simulink model "Scenario_PTF_path_following_v1"  (R2024b)
settings: Solver=ode1  StartTime=0.0  StopTime=1000  FixedStep=.05  RelTol=1e-3  EnableMultiTasking=on
InitFcn:
  | omega_n = 1; r_limit = 10; scale = 1;
values from neighbouring files (symbols this model uses):
  complete_Cx = B_fine * control_points    [MCM_v4.m]
  complete_DCx = B_fine * control_points_deriv    [MCM_v4.m]
  complete_time = [complete_time(1:end-1,:); segment_time_shifted']    [MCM_v4.m]
libraries: simulink x5
settings Model: Creator=isaackaminer  LastModifiedBy=bradenzukowski
settings SolverCC: AlgebraicLoopSolver=TrustRegion
settings DataIOCC: LimitDataPoints=on  SaveFormat=StructureWithTime  SignalLoggingSaveFormat=ModelDataLogs  ReturnWorkspaceOutputs=off
settings OptimizationCC: BlockReduction=off  DefaultParameterBehavior=Inlined  BufferReuse=off  LifeSpan=inf
settings DebuggingCC: SolverPrmCheckMsg=warning  MultiTaskDSMMsg=warning  MultiTaskCondExecSysMsg=none  UnconnectedInputMsg=warning  UnconnectedOutputMsg=warning  UnconnectedLineMsg=warning  InitInArrayFormatMsg=none  SFUnexpectedBacktrackingDiag=warning  SFNoUnconditionalDefaultTransitionDiag=warning  SFExecutionAtInitializationDiag=none  ArithmeticOperatorsInVariantConditions=warning
settings HardwareCC: ProdBitPerPointer=32  ProdBitPerSizeT=32  ProdBitPerPtrDiffT=32  ProdLargestAtomicFloat=None  ProdIntDivRoundTo=Undefined  ProdEndianess=Unspecified  ProdWordSize=32  ProdHWDeviceType=32-bit Generic
settings ModelReferenceCC: EnableRefExpFcnMdlSchedulingChecks=on  PropagateSignalLabelsOutOfModel=off
settings SFSimCC: SimUseLocalCustomCode=off  CustomCodeUndefinedFunction=UseInterfaceOnly
settings RTWCC: RTWUseLocalCustomCode=off  GPUComputeCapability=3.5
settings CodeAppCC: StateflowObjectComments=on
settings GRTTargetCC: TargetLangStandard=C89/C90 (ANSI)
settings ConfigComp: CovMetricSettings=dw  CovSaveCumulativeToWorkspaceVar=on  CovSaveSingleToWorkspaceVar=on  CovExternalEMLEnable=off

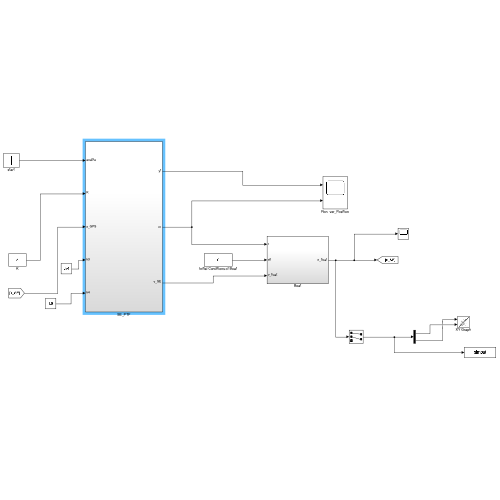
[thumbnail: Simulink's stored preview of the top-level diagram]
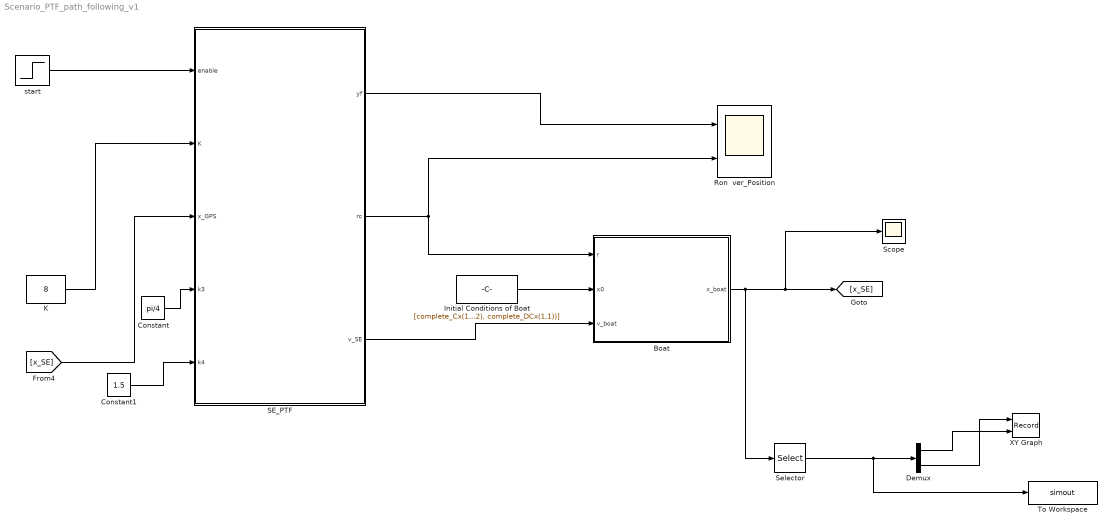
== system Scenario_PTF_path_following_v1 ==
  Boat : Subsystem
  Constant : Constant  Value=pi/4
  Constant1 : Constant  Value=1.5
  Demux : Demux  Outputs=2
  Initial Conditions of Boat : Constant  Value=[complete_Cx(1,1);complete_Cx(1,2);atan2(complete_DCx(1,2), complete_DCx(1,1))]
  K : Constant  Value=8
  Ron  ver_Position : Scope  NumInputPorts=2
  SE_PTF : Subsystem
  Scope : Scope
  Selector : Selector  InputPortWidth=3  IndexOptions=Index vector (dialog)  Indices=[1 2]  OutputSizes=1
  To Workspace : ToWorkspace  VariableName=simout  SaveFormat=Timeseries  SampleTime=-1
  XY Graph : Record  FileSettingsInternal="{\"entries\":[{\"content\":{\"excelSettings\":{\"content\":{},\"type\":\"Streamout.ExcelSettings\"}},\"type\":\"Streamout.FileSettingStorage\",\"uuid\":\"\"}],\"packageUris\":[\"http:\\/\\/schema.mathworks.com\\/mf0\\/streamout_blocks\\/R2020a\"],\"version\":\"1.0\"}"  Layout=[1 1]  SignalsInternal="{\"entries\":[{\"content\":{\"signals\":[{\"content\":{\"blockPath\":[],\"dimensions\":[1],\"domain\":\"\",\"lineColor\":\"#a2142f\",\"plots\":[ 1 ],\"port\":1,\"sid\":[\"\"],\"signalID\":1,\"signalName\":\"Demux:2\"},\"type\":\"RecordBlkView.Signal\",\"uuid\":\"\"},{\"content\":{\"blockPath\":[],\"dimensions\":[1],\"domain\":\"\",\"lineColor\":\"#139fff\",\"plots\":[ 1 ],\"port\":2,\"sid\":[\"\"],\"signalID\":2,\"signalName\":\"Demux:1\"},\"type\":\"RecordBlkView.Signal\",\"uuid\":\"\"}]},\"type\":\"RecordBlkView.InputSignals\",\"uuid\":\"\"}],\"packageUris\":[\"http:\\/\\/schema.mathworks.com\\/mf0\\/streamout_blocks\\/R2020a\"],\"version\":\"1.0\"}"  VisualizationBindings="{\"xyplotplugin\":{\"info\":[{\"series\":[{\"bindingParametersList\":[{\"parameter\":\"X-Axis\",\"signalID\":1,\"signalName\":\"Demux:2\"},{\"parameter\":\"Y-Axis\",\"signalID\":2,\"signalName\":\"Demux:1\"}],\"seriesID\":0}],\"subplotID\":1}]}}"  CompatibilityTag=XY
  start : Step  Time=0  SampleTime=0
  wires:
  start/1 -> SE_PTF/1(enable)
  SE_PTF/2(rc) -> Boat/1(r), Ron  ver_Position/2
  [x_SE] -> SE_PTF/3(x_GPS)
  SE_PTF/1(yf) -> Ron  ver_Position/1
  Demux/2 -> XY Graph/1
  Boat/1(x_boat) -> Scope/1, [x_SE], Selector/1
  Initial Conditions of Boat/1 -> Boat/2(x0)
  Selector/1 -> To Workspace/1, Demux/1
  Demux/1 -> XY Graph/2
  K/1 -> SE_PTF/2(K)
  Constant/1 -> SE_PTF/4(k3)
  Constant1/1 -> SE_PTF/5(k4)
  SE_PTF/3(v_SE) -> Boat/3(v_boat)

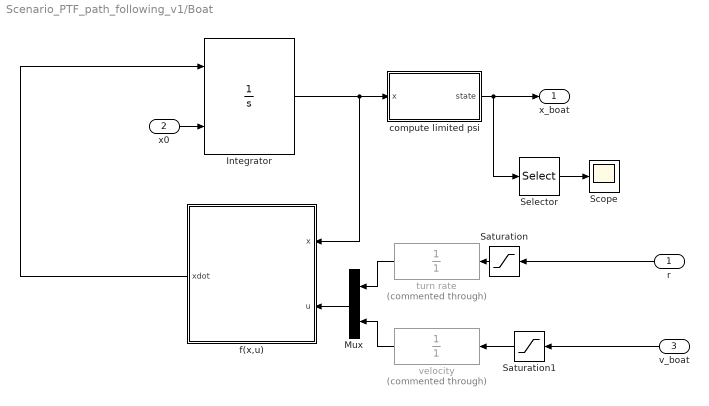
== system Scenario_PTF_path_following_v1/Boat ==
  r : Inport
  x0 : Inport  Port=2
  v_boat : Inport  Port=3
  Integrator : Integrator  InitialConditionSource=external
  Mux : Mux  Inputs=2
  Saturation : Saturate  UpperLimit=.5  LowerLimit=-.5
  Saturation1 : Saturate  UpperLimit=3  LowerLimit=0
  Scope : Scope
  Selector : Selector  InputPortWidth=3  IndexOptions=Index vector (dialog)  Indices=3  OutputSizes=1
  compute limited psi : MATLAB Function  TreatAsAtomicUnit=on
  f(x,u) : MATLAB Function  TreatAsAtomicUnit=on
  turn rate : TransferFcn  Commented=through  Denominator=[1]
  velocity : TransferFcn  Commented=through  Denominator=[1]
  x_boat : Outport  VectorParamsAs1DForOutWhenUnconnected=off
  wires:
  f(x,u)/1(xdot) -> Integrator/1
  x0/1 -> Integrator/2
  Integrator/1 -> compute limited psi/1(x), f(x,u)/1(x)
  compute limited psi/1(state) -> Selector/1, x_boat/1
  turn rate/1 -> Mux/1
  Mux/1 -> f(x,u)/2(u)
  Selector/1 -> Scope/1
  velocity/1 -> Mux/2
  Saturation/1 -> turn rate/1
  r/1 -> Saturation/1
  Saturation1/1 -> velocity/1
  v_boat/1 -> Saturation1/1

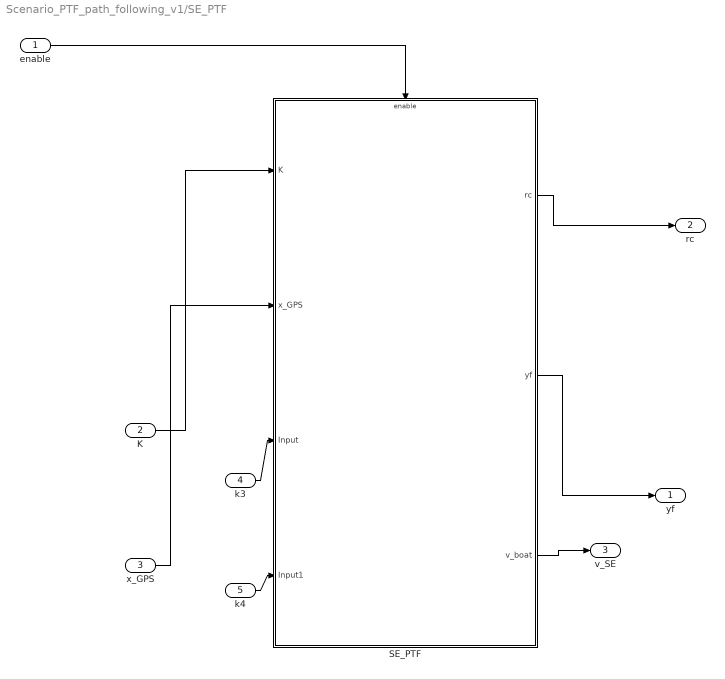
== system Scenario_PTF_path_following_v1/SE_PTF ==
  enable : Inport
  K : Inport  Port=2
  x_GPS : Inport  Port=3
  k3 : Inport  Port=4
  k4 : Inport  Port=5
  SE_PTF : Subsystem
  yf : Outport  VectorParamsAs1DForOutWhenUnconnected=off
  rc : Outport  Port=2  VectorParamsAs1DForOutWhenUnconnected=off
  v_SE : Outport  Port=3
  wires:
  K/1 -> SE_PTF/1(K)
  SE_PTF/2(yf) -> yf/1
  enable/1 -> SE_PTF/Enable
  x_GPS/1 -> SE_PTF/2(x_GPS)
  SE_PTF/1(rc) -> rc/1
  k3/1 -> SE_PTF/3(Input)
  k4/1 -> SE_PTF/4(Input1)
  SE_PTF/3(v_boat) -> v_SE/1

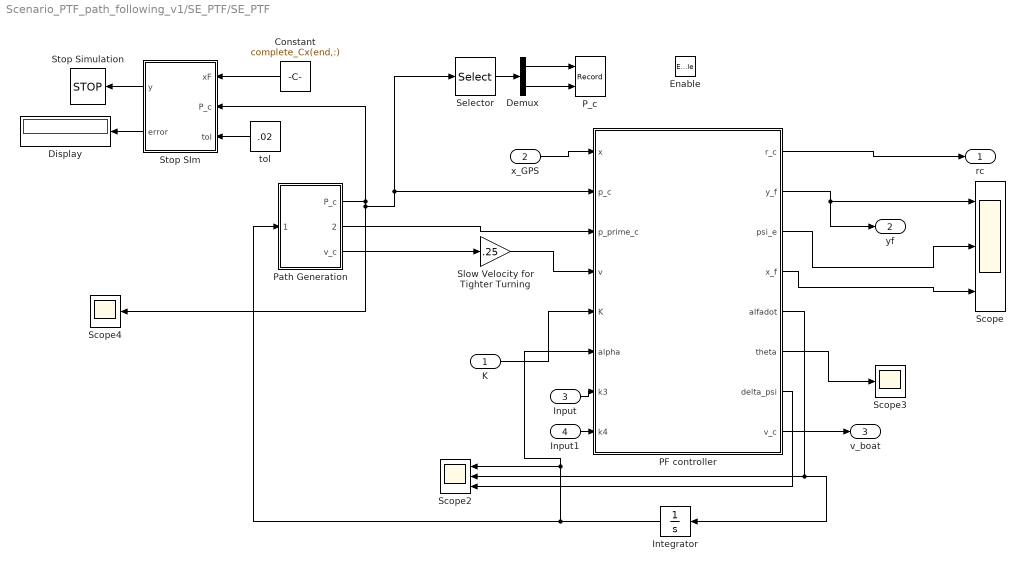
== system Scenario_PTF_path_following_v1/SE_PTF/SE_PTF ==
  K : Inport
  x_GPS : Inport  Port=2
  Input : Inport  Port=3
  Input1 : Inport  Port=4
  Enable : EnablePort  PropagateVarSize=During execution
  Constant : Constant  Value=complete_Cx(end,:)
  Demux : Demux  Outputs=2
  Display : Display
  Integrator : Integrator
  PF controller : MATLAB Function  TreatAsAtomicUnit=on
  P_c : Record  FileSettingsInternal="{\"entries\":[{\"content\":{\"excelSettings\":{\"content\":{},\"type\":\"Streamout.ExcelSettings\"}},\"type\":\"Streamout.FileSettingStorage\",\"uuid\":\"\"}],\"packageUris\":[\"http:\\/\\/schema.mathworks.com\\/mf0\\/streamout_blocks\\/R2020a\"],\"version\":\"1.0\"}"  Layout=[1 1]  SignalsInternal="{\"entries\":[{\"content\":{\"signals\":[{\"content\":{\"blockPath\":[],\"dimensions\":[1],\"domain\":\"\",\"lineColor\":\"#a2142f\",\"plots\":[ 1 ],\"port\":1,\"sid\":[\"\"],\"signalID\":1,\"signalName\":\"Demux:1\"},\"type\":\"RecordBlkView.Signal\",\"uuid\":\"\"},{\"content\":{\"blockPath\":[],\"dimensions\":[1],\"domain\":\"\",\"lineColor\":\"#139fff\",\"plots\":[ 1 ],\"port\":2,\"sid\":[\"\"],\"signalID\":2,\"signalName\":\"Demux:2\"},\"type\":\"RecordBlkView.Signal\",\"uuid\":\"\"}]},\"type\":\"RecordBlkView.InputSignals\",\"uuid\":\"\"}],\"packageUris\":[\"http:\\/\\/schema.mathworks.com\\/mf0\\/streamout_blocks\\/R2020a\"],\"version\":\"1.0\"}"  VisualizationBindings="{\"xyplotplugin\":{\"info\":[{\"series\":[{\"bindingParametersList\":[{\"parameter\":\"X-Axis\",\"signalID\":1,\"signalName\":\"Demux:1\"},{\"parameter\":\"Y-Axis\",\"signalID\":2,\"signalName\":\"Demux:2\"}],\"seriesID\":0}],\"subplotID\":1}]}}"  CompatibilityTag=XY  st=-1
  Path Generation : Subsystem
  Scope : Scope  NumInputPorts=3
  Scope2 : Scope  NumInputPorts=3
  Scope3 : Scope
  Scope4 : Scope
  Selector : Selector  InputPortWidth=3  IndexOptions=Index vector (dialog)  Indices=[2 1]  OutputSizes=1
  Slow Velocity for Tighter Turning : Gain  Gain=.25
  Stop SIm : MATLAB Function  TreatAsAtomicUnit=on
  Stop Simulation : Stop
  tol : Constant  Value=.02
  rc : Outport  VectorParamsAs1DForOutWhenUnconnected=off
  yf : Outport  Port=2  VectorParamsAs1DForOutWhenUnconnected=off
  v_boat : Outport  Port=3
  wires:
  x_GPS/1 -> PF controller/1(x)
  Path Generation/2(P_dot_c) -> PF controller/3(p_prime_c)
  Path Generation/1(P_c) -> Scope4/1, Selector/1, PF controller/2(p_c), Stop SIm/2(P_c)
  PF controller/2(y_f) -> Scope/1, yf/1
  PF controller/1(r_c) -> rc/1
  K/1 -> PF controller/5(K)
  PF controller/5(alfadot) -> Integrator/1, Scope2/2
  PF controller/3(psi_e) -> Scope/2
  PF controller/4(x_f) -> Scope/3
  PF controller/6(theta) -> Scope3/1
  PF controller/7(delta_psi) -> Scope2/3
  Selector/1 -> Demux/1
  Demux/1 -> P_c/1
  Demux/2 -> P_c/2
  Integrator/1 -> Scope2/1, PF controller/6(alpha), Path Generation/1(alpha)
  Stop SIm/1(y) -> Stop Simulation/1
  Constant/1 -> Stop SIm/1(xF)
  tol/1 -> Stop SIm/3(tol)
  Stop SIm/2(error) -> Display/1
  Input/1 -> PF controller/7(k3)
  Input1/1 -> PF controller/8(k4)
  PF controller/8(v_c) -> v_boat/1
  Path Generation/3(v_c) -> Slow Velocity for Tighter Turning/1
  Slow Velocity for Tighter Turning/1 -> PF controller/4(v)

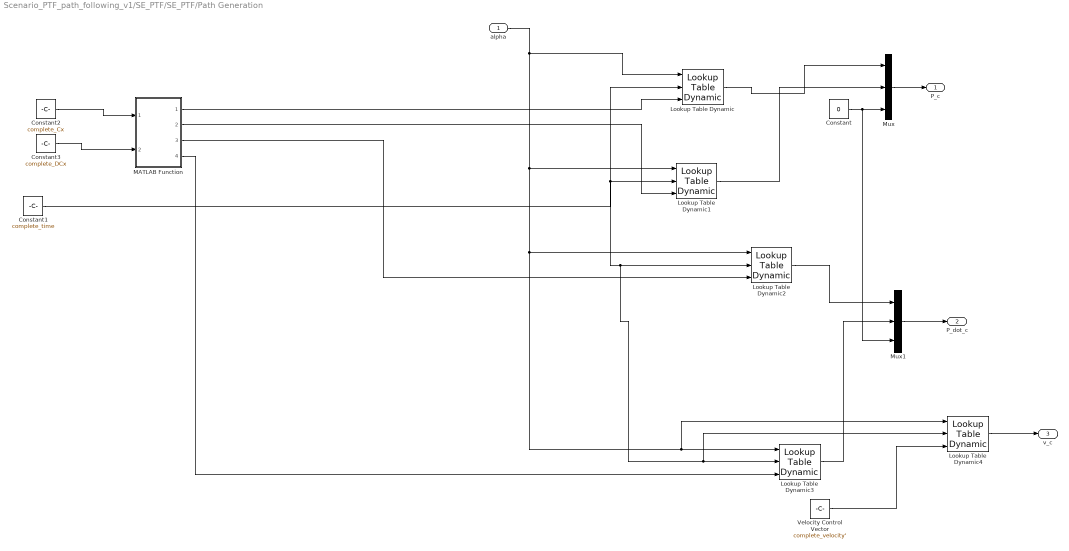
== system Scenario_PTF_path_following_v1/SE_PTF/SE_PTF/Path Generation ==
  alpha : Inport
  Constant : Constant  Value=0
  Constant1 : Constant  Value=complete_time
  Constant2 : Constant  Value=complete_Cx
  Constant3 : Constant  Value=complete_DCx
  Lookup Table Dynamic{,1..4} (5 alike) : simulink/Lookup Tables/Lookup Table Dynamic  LookUpMeth=Interpolation-Use End Values  OutDataType=fixdt('double')  OutScaling=[]  OutputDataTypeScalingMode=Specify via dialog  OutDataTypeStr=double  DoSatur=off
  MATLAB Function : MATLAB Function  TreatAsAtomicUnit=on
  Mux : Mux  Inputs=3
  Mux1 : Mux  Inputs=3
  Velocity Control Vector : Constant  Value=complete_velocity'
  P_c : Outport  PortDimensions=3
  P_dot_c : Outport  Port=2  PortDimensions=3
  v_c : Outport  Port=3
  wires:
  Lookup Table Dynamic/1 -> Mux/1
  Lookup Table Dynamic1/1 -> Mux/2
  Mux/1 -> P_c/1
  Mux1/1 -> P_dot_c/1
  Lookup Table Dynamic2/1 -> Mux1/1
  Lookup Table Dynamic3/1 -> Mux1/2
  MATLAB Function/1(XN_trans) -> Lookup Table Dynamic/3
  MATLAB Function/2(YN_trans) -> Lookup Table Dynamic1/3
  MATLAB Function/4(DYN_trans) -> Lookup Table Dynamic3/3
  MATLAB Function/3(DXN_trans) -> Lookup Table Dynamic2/3
  Constant2/1 -> MATLAB Function/1(Cx_traj)
  Constant3/1 -> MATLAB Function/2(DCx_traj)
  alpha/1 -> Lookup Table Dynamic/1, Lookup Table Dynamic4/1, Lookup Table Dynamic3/1, Lookup Table Dynamic2/1, Lookup Table Dynamic1/1
  Constant/1 -> Mux1/3, Mux/3
  Constant1/1 -> Lookup Table Dynamic/2, Lookup Table Dynamic4/2, Lookup Table Dynamic3/2, Lookup Table Dynamic2/2, Lookup Table Dynamic1/2
  Velocity Control Vector/1 -> Lookup Table Dynamic4/3
  Lookup Table Dynamic4/1 -> v_c/1

== matlab function Scenario_PTF_path_following_v1/SE_PTF/SE_PTF/PF controller ==
  settings: updateMethod=DISCRETE
  data: x input; r_c output; p_c input; p_prime_c input; v input; K input; y_f output; psi_e output; x_f output; alfadot output; alpha input; theta output; delta_psi output; k3 input; k4 input; v_c output
 function [r_c,y_f,psi_e,x_f,alfadot,theta,delta_psi,v_c]  = fcn(x,p_c,p_prime_c,v,K,alpha,k3,k4)
%#codegen

persistent T0 N10 N20 alpha0

if isempty(T0)
    T0 = [1;0;0]; 
end

if isempty(N20)
    N20 = [0;0;1];
end

if isempty(N10)
    N10 = [0;1;0];
end
if isempty(alpha0)
    alpha0 = 0;
end

v_c = v;

% Sub parameters

% x = [psi x y]

p_rover = [x(1:2);0];
psi = x(3);

% compute nearest point on the circle
% i = (p_rover - p_center)/norm(p_rover - p_center);
% 
% p_c = p_center + R*i;
%  
% alpha = atan2(p_c(2) - p_center(2), p_c(1) - p_center(1));


% p_c = p_center + R*[(alpha); sin(omega*alpha);0]; % commanded position 
% p_prime_c = R*[1; omega*cos(omega*alpha);0];
% T = [1;omega*cos(omega*alpha);0]/norm([1;omega*cos(omega*alpha);0]);

T = p_prime_c/norm(p_prime_c);
T = T/norm(T);

% PTF implementation
%     B1 = cross(T,T0);
    B1 = cross(T0,T);
    if norm(B1) == 0 
        N1 = N10; 
        N2 = cross(T,N1);
        theta = 0;
        k1 = 0; 
        k2 = 0;
    else 
        B1 = B1/norm(B1);
        if T'*T0 > 1
            theta = acos(1);
        elseif T'*T0 < -1
            theta = acos(-1);
        else
            theta = acos(T'*T0);
        end
        
        N1 = rodrigues_rot(N10,B1,theta); % sinusoid and circle
        N1 = N1/norm(N1);
        N2 = cross(T,N1)/norm(cross(T,N1));
        ds_dalpha = norm(p_prime_c); 
        if abs(alpha-alpha0) == 0
            k1 = 0; 
            k2 = 0;
        else
            k1 = norm(N1 - N10)/abs(alpha-alpha0)/ds_dalpha;
            k2 = norm(N2 - N20)/abs(alpha-alpha0)/ds_dalpha;
        end
    end
    
T0 = T; N10 = N1; N20 = N2; alpha0 = alpha; R0 = 1/(k1+eps);
 
R_I2F = [T N1 N2]'; 

psi_F = atan2(T(2),T(1));
psi_e = wrapToPi(psi_F - psi); 
% 
pe_F = R_I2F*(p_c - p_rover);
x_f = pe_F(1);
y_f = pe_F(2);
%
sdot = (v*cos(psi_e) - 2*K*x_f);
sdot = max(sdot, 0);
delta_psi = -k3 * tanh(k4 * y_f);
ydot = v * sin(psi_e);
delta_psi_dot = -k3 * k4 * (1 - tanh(k4 * y_f)^2) * ydot;

% y_f_dot = v*sin(psi_e);
% delta_psi_dot = -(1/(d + abs(y_f)) + 1e-8*(y_f*sign(y_f))/(d + abs(y_f))^2)/(1 - y_f^2/(d + abs(y_f))^2)^(1/2)*y_f_dot;
% % mysinc = (sin(psi_e) - sin(delta_psi))/(psi_e - delta_psi);
% mysinc = cos((psi_e + delta_psi)/2)*sinc((psi_e - delta_psi)/2);
% 
% r_c = k1*sdot + delta_psi_dot - y_f*v*mysinc + K*(psi_e - delta_psi);

%r_c = k1*sdot   + K*(psi_e - delta_psi);
r_c = k1 * sdot + delta_psi_dot + K * (psi_e - delta_psi);
alfadot = sdot / norm(p_prime_c);
% alfadot = 1;
end

% rodrigues_rot - Rotates array of 3D vectors by an angle theta about vector k.
% Direction is determined by the right-hand (screw) rule.
%
% Syntax:  v_rot = rodrigues(v,k,theta)
%
% Inputs:
%    v - Array of three dimensional vectors to rotate. Array can be 
%           composed of N rows of 3D row vectors or N columns of 3D column
%           vectors. If v is 3x3 array, it is assumed that it is 3 rows of
%           3 3D row vectors.
%    k - Rotation axis (does not need to be unit vector)
%    theta - Rotation angle in radians; positive according to right-hand
%           (screw) rule
%
%   Note: k and individual 3D vectors in v array must be same orientation.
%           
%
% Outputs:
%    v_rot - Array of rotated vectors.
%
% Other m-files required: dot.m (built-in MATLAB)
% Subfunctions: none
% MAT-files required: none
%
% Author: Ismail Hameduddin
%           Mechanical Engineering, Purdue University
% email: ihameduddin@gmail.com
% Website: http://www.ismailh.com
% January 2011; Last revision: 2-January-2012

%------------- BEGIN CODE --------------

function v_rot = rodrigues_rot(v,k,theta)
    [m,n] = size(v);
%     if (m ~= 3 && n ~= 3)
%         error('input vector is/are not three dimensional'), end
%     if (size(v) ~= size(k)) 
%         error('rotation vector v and axis k have different dimensions'),end
    
    k = k/sqrt(k(1)^2 + k(2)^2 + k(3)^2); % normalize rotation axis
    No = numel(v)/3; % number of vectors in array
    v_rot = v; % initialize rotated vector array
    if ( n == 3 )
        crosskv = v(1,:); % initialize cross product k and v with right dim.
        for i = 1:No
            crosskv(1) = k(2)*v(i,3) - k(3)*v(i,2);
            crosskv(2) = k(3)*v(i,1) - k(1)*v(i,3); 
            crosskv(3) = k(1)*v(i,2) - k(2)*v(i,1);
            v_rot(i,:) = cos(theta)*v(i,:) + (crosskv)*sin(theta)...
                            + k*(dot(k,v(i,:)))*(1 - cos(theta));
        end
    else % if m == 3 && n ~= 3
        crosskv = v(:,1); % initialize cross product k and v with right dim.
        for i = 1:No
            crosskv(1) = k(2)*v(3,i) - k(3)*v(2,i);
            crosskv(2) = k(3)*v(1,i) - k(1)*v(3,i); 
            crosskv(3) = k(1)*v(2,i) - k(2)*v(1,i);
            v_rot(:,i) = cos(theta)*v(:,i) + (crosskv)*sin(theta)...
                            + k*(dot(k,v(:,i)))*(1 - cos(theta));
        end
    end
end

== matlab function Scenario_PTF_path_following_v1/Boat/compute limited psi ==
  data: x input; state output
function state  = fcn(x)
%#codegen

% Sub parameters

% x = [psi x y]

psi_in = x(3);
psi = atan2(sin(psi_in),cos(psi_in));
state = [x(1:2);psi];

== matlab function Scenario_PTF_path_following_v1/SE_PTF/SE_PTF/Stop SIm ==
  data: xF input; y output; P_c input; tol input; error output
function [y,error] = fcn(xF,P_c,tol)

if norm(xF(1:2) - P_c(1:2)) <= tol
    y = 1;
else 
    y = 0
end

error = norm(xF(1:2) - P_c(1:2));

== matlab function Scenario_PTF_path_following_v1/SE_PTF/SE_PTF/Path Generation/MATLAB Function ==
  data: Cx_traj input; XN_trans output; YN_trans output; DXN_trans output; DYN_trans output; DCx_traj input
function [XN_trans, YN_trans, DXN_trans, DYN_trans] = extractTrajectoryColumns(Cx_traj, DCx_traj)
XN_trans = Cx_traj(:,1)';  
YN_trans = Cx_traj(:,2)';  
DXN_trans = DCx_traj(:,1)';  
DYN_trans = DCx_traj(:,2)';
end

== matlab function Scenario_PTF_path_following_v1/Boat/f(x,u) ==
  data: x input; xdot output; u input
function xdot   = fcn(x,u)
%#codegen

% Sub parameters

% x = [psi x y]
% u = [r v]

psi = x(3); 

r = u(1); v = u(2);

xdot = [v*cos(psi);
       v*sin(psi); 
                r];

       
   
% psi0 = atan2(xdot(2),xdot(1));
